simulink model "temperature_control"  (R2023a)
settings: Solver=VariableStepAuto  StartTime=0.0  StopTime=10.0  RelTol=1e-3
values from neighbouring files (symbols this model uses):
  Ku = 3    [script.m]
  taw = 30    [script.m]
settings Model: Creator=eslam  LastModifiedBy=eslam

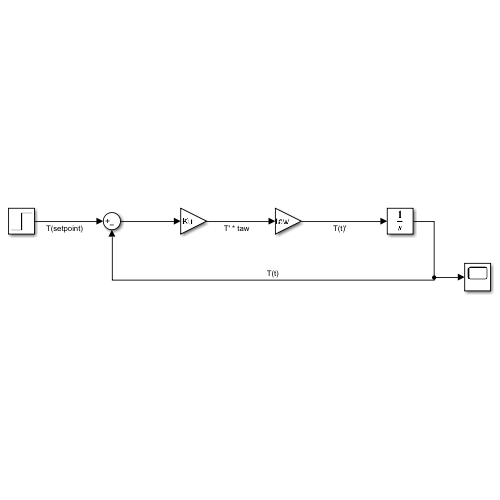
[thumbnail: Simulink's stored preview of the top-level diagram]
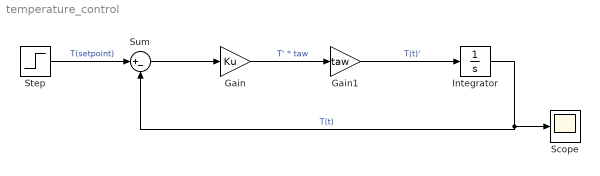
== system temperature_control ==
  Gain : Gain  Gain=Ku
  Gain1 : Gain  Gain=taw
  Integrator : Integrator
  Scope : Scope
  Step : Step  SampleTime=0
  Sum : Sum  Inputs=|+-
  wires:
  Step/1 -> Sum/1  "T(setpoint)"
  Sum/1 -> Gain/1
  Gain/1 -> Gain1/1  "T' * taw"
  Gain1/1 -> Integrator/1  "T(t)'"
  Integrator/1 -> Scope/1, Sum/2  "T(t)"
